simulink model "Boost_Simulated_calibration"  (R2023b)
settings: Solver=VariableStepAuto  StartTime=0.0  StopTime=0.1  RelTol=1e-3
libraries: spsSeriesRLCBranchLib x5, spsCurrentMeasurementLib x4, spsMosfetLib x2, spsDCVoltageSourceLib x1, simulink x1, spsVoltageMeasurementLib x1, spspowerguiLib x1
settings Model: Creator=23227  LastModifiedBy=23227

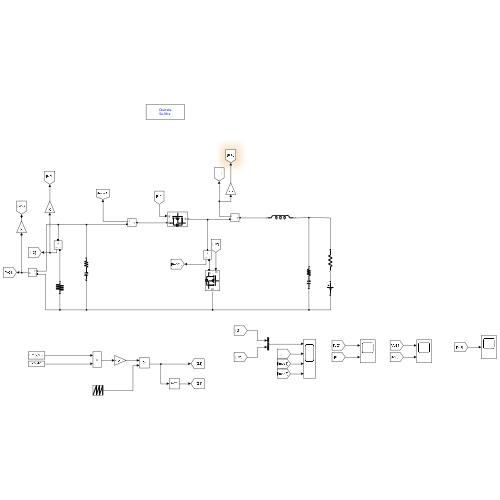
[thumbnail: Simulink's stored preview of the top-level diagram]
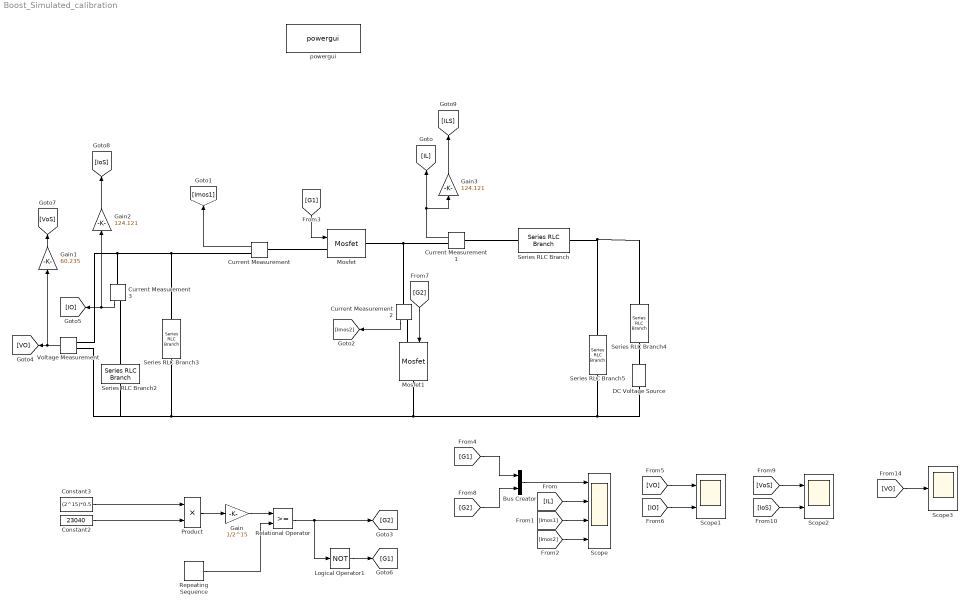
== system Boost_Simulated_calibration ==
  Bus Creator : BusCreator  Inputs=2
  Constant2 : Constant  Value=23040
  Constant3 : Constant  Value=(2^15)*0.5
  Current Measurement{,1..3} (4 alike) : spsCurrentMeasurementLib/Current Measurement  PhasorSimulation=off  OutputType=Complex  PSBequivalent=0
  DC Voltage Source : spsDCVoltageSourceLib/DC Voltage Source  Amplitude=24  Measurements=None
  Gain : Gain  Gain=1/2^15
  Gain1 : Gain  Gain=60.235
  Gain2 : Gain  Gain=124.121
  Gain3 : Gain  Gain=124.121
  Logical Operator1 : Logic  Operator=NOT  AllPortsSameDT=off  OutDataTypeStr=boolean
  Mosfet : spsMosfetLib/Mosfet  Ron=0.007  Lon=0  Rd=0.01  Vfd=0  IC=0  Rs=1e5  Cs=inf  Measurements=off
  Mosfet1 : spsMosfetLib/Mosfet  Ron=0.007  Lon=0  Rd=0.01  Vfd=0  IC=0  Rs=1e5  Cs=inf  Measurements=off
  Product : Product
  Relational Operator : RelationalOperator  OutDataTypeStr=boolean  RndMeth=Simplest  InputSameDT=off
  Repeating Sequence : simulink/Sources/Repeating Sequence  rep_seq_t=[0 1/200e3]  rep_seq_y=[0 23040]
  Scope : Scope  NumInputPorts=4
  Scope1 : Scope  NumInputPorts=2
  Scope2 : Scope  NumInputPorts=2
  Scope3 : Scope
  Series RLC Branch : spsSeriesRLCBranchLib/Series RLC Branch  LConnTagsString=__new0  RConnTagsString=__new0  BranchType=L  Resistance=1  Inductance=22e-6  SetiL0=off  InitialCurrent=0  Capacitance=1e-6  Setx0=off  InitialVoltage=0  Measurements=None
  Series RLC Branch2 : spsSeriesRLCBranchLib/Series RLC Branch  LConnTagsString=__new0  RConnTagsString=__new0  BranchType=R  Resistance=9.6  Inductance=1e-3  SetiL0=off  InitialCurrent=0  Capacitance=1e-6  Setx0=off  InitialVoltage=0  Measurements=None
  Series RLC Branch3 : spsSeriesRLCBranchLib/Series RLC Branch  LConnTagsString=__new0  RConnTagsString=__new0  BranchType=RC  Resistance=2E-3  Inductance=1e-3  SetiL0=off  InitialCurrent=0  Capacitance=4.08e-3  Setx0=on  InitialVoltage=24  Measurements=None
  Series RLC Branch4 : spsSeriesRLCBranchLib/Series RLC Branch  LConnTagsString=__new0  RConnTagsString=__new0  BranchType=R  Resistance=0.000001  Inductance=1e-3  SetiL0=off  InitialCurrent=0  Capacitance=1e-3  Setx0=off  InitialVoltage=0  Measurements=None
  Series RLC Branch5 : spsSeriesRLCBranchLib/Series RLC Branch  LConnTagsString=__new0  RConnTagsString=__new0  BranchType=RC  Resistance=2E-3  Inductance=1e-3  SetiL0=off  InitialCurrent=0  Capacitance=4.08e-3  Setx0=off  InitialVoltage=24  Measurements=None
  Voltage Measurement : spsVoltageMeasurementLib/Voltage Measurement  PhasorSimulation=off  OutputType=Complex  PSBequivalent=0
  powergui : spspowerguiLib/powergui  Priority=1  SimulationMode=Discrete  SampleTime=5e-8  frequency=60  Iterations=50  frequencyindice=0  Pbase=100e6  ErrMax=1e-4  UnitsV=kV  UnitsW=MW  buscounter=0  FunctionMessages=off  echomessages=off  EnableUseOfTLC=off  CurrentSourceSwitches=off  DisableSnubberDevices=off  DisableRonSwitches=off  DisableVfSwitches=off  DisplayEquations=off  AutomaticDiscreteSolvers=off  SolverType=Tustin/Backward Euler (TBE)  Interpol=off  ExternalGateDelay=off  methode=off  Ts=10  x0status=blocks  SPID=off  SwTol=0  HookPort=off  NonlinearTolerance=1e-4  nMaxIteration=100  ContinueOnMaxIteration=off  RestoreLinks=warning  ResistiveCurrentMeasurement=off  Frange=[0:2:500]  Ylog=off  Xlog=on  ShowGrid=off  save=off  variable=ZData  structure=0  ZoomFFT=off  StartTime=0.0  cycles=1  DisplayStyle=1  fundamental=60  FreqAxis=off  MaxFrequency=1000  frequencyindicesteady=1  RmsSteady=1  display=off
  wires:
  [VoS] -> Scope2/1
  Constant2/1 -> Product/2
  [G1] -> Mosfet/1
  [VO] -> Scope3/1
  Current Measurement/1 -> [Imos1]
  Current Measurement2/1 -> [Imos2]
  [IoS] -> Scope2/2
  Gain1/1 -> [VoS]
  [G1] -> Bus Creator/1
  [VO] -> Scope1/1
  Gain2/1 -> [IoS]
  Relational Operator/1 -> [G2], Logical Operator1/1
  [G2] -> Mosfet1/1
  Repeating Sequence/1 -> Relational Operator/2
  [IL] -> Scope/2
  [IO] -> Scope1/2
  Product/1 -> Gain/1
  Bus Creator/1 -> Scope/1
  [Imos1] -> Scope/3
  Voltage Measurement/1 -> [VO], Gain1/1
  [Imos2] -> Scope/4
  Constant3/1 -> Product/1
  Gain/1 -> Relational Operator/1
  [G2] -> Bus Creator/2
  Current Measurement3/1 -> [IO], Gain2/1
  Logical Operator1/1 -> [G1]
  Current Measurement1/1 -> Gain3/1, [IL]
  Gain3/1 -> [ILS]
  connections:
  Series RLC Branch3/LConn1 -- Current Measurement/RConn1 -- Current Measurement3/LConn1 -- Voltage Measurement/LConn1
  Current Measurement1/RConn1 -- Current Measurement2/LConn1 -- Mosfet/RConn1
  Series RLC Branch4/RConn1 -- DC Voltage Source/RConn1
  Current Measurement3/RConn1 -- Series RLC Branch2/LConn1
  Series RLC Branch3/RConn1 -- Series RLC Branch2/RConn1 -- Voltage Measurement/LConn2 -- Mosfet1/RConn1 -- Series RLC Branch5/RConn1 -- DC Voltage Source/LConn1
  Series RLC Branch/LConn1 -- Current Measurement1/LConn1
  Mosfet1/LConn1 -- Current Measurement2/RConn1
  Current Measurement/LConn1 -- Mosfet/LConn1
  Series RLC Branch5/LConn1 -- Series RLC Branch4/LConn1 -- Series RLC Branch/RConn1
